simulink model "PowE_lab4_3"  (R2021b)
settings: Solver=VariableStepAuto  StartTime=0.0  StopTime=0.06  RelTol=1e-3
libraries: spsDetailedThyristorLib x2, spsACVoltageSourceLib x1, spsCurrentMeasurementLib x1, spsLinearTransformerLib x1, spsMeanLib x1, spsRMSLib x1, spsSeriesRLCBranchLib x1, spsVoltageMeasurementLib x1, spspowerguiLib x1
settings Model: Creator=shrey  LastModifiedBy=Asus

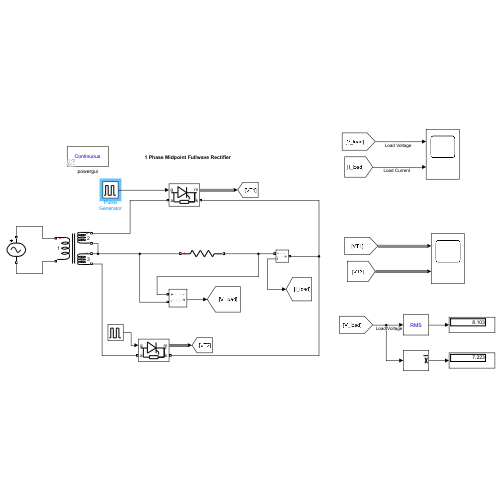
[thumbnail: Simulink's stored preview of the top-level diagram]
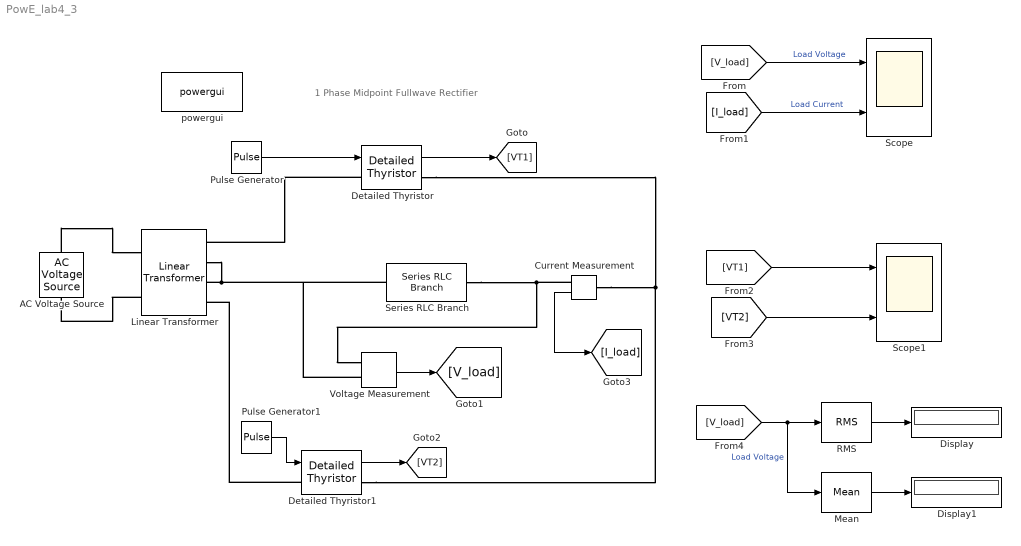
== system PowE_lab4_3 ==
  note: 1 Phase Midpoint Fullwave Rectifier
  AC Voltage Source : spsACVoltageSourceLib/AC Voltage Source  Amplitude=230  Phase=0  Frequency=50  SampleTime=0  Measurements=None  BusType=swing  Pref=10e3  Qref=0  Qmin=-inf  Qmax=+inf
  Current Measurement : spsCurrentMeasurementLib/Current Measurement  PhasorSimulation=off  OutputType=Complex  PSBequivalent=0
  Detailed Thyristor : spsDetailedThyristorLib/Detailed Thyristor  Ron=0.001  Lon=1e-3  Vf=0.8  IL=0.1  Tq=100e-6  IC=0  Rs=500  Cs=250e-9  Measurements=on
      settings: SourceProductBaseCode=PS
  Detailed Thyristor1 : spsDetailedThyristorLib/Detailed Thyristor  Ron=0.001  Lon=1e-3  Vf=0.8  IL=0.1  Tq=100e-6  IC=0  Rs=500  Cs=250e-9  Measurements=on
      settings: SourceProductBaseCode=PS
  Display : Display
  Display1 : Display
  Linear Transformer : spsLinearTransformerLib/Linear Transformer  UNITS=pu  NominalPower=[ 250e6 60 ]  winding1="[ 230  0.002  0.08 ]"  winding2="[ 12  0.002  0.0 ]"  ThreeWindings=on  winding3=[ 12 0.002 0.0 ]  RmLm=[ 500 500 ]  Measurements=None  DataType=off
  Mean : spsMeanLib/Mean  Freq=60  Vinit=0  Ts=0
  Pulse Generator : DiscretePulseGenerator  PulseType=Time based  Period=0.02  PulseWidth=5  PhaseDelay=0.02*(0/360)
  Pulse Generator1 : DiscretePulseGenerator  PulseType=Time based  Period=10  PulseWidth=5  PhaseDelay=0.02*(180)/360
  RMS : spsRMSLib/RMS  TrueRMS=on  Freq=60  RMSInit=120  Ts=0
  Scope : Scope  NumInputPorts=2
  Scope1 : Scope  NumInputPorts=2
  Series RLC Branch : spsSeriesRLCBranchLib/Series RLC Branch  LConnTagsString=__new0  RConnTagsString=__new0  BranchType=R  Resistance=100  Inductance=1e-3  SetiL0=off  InitialCurrent=0  Capacitance=1e-6  Setx0=off  InitialVoltage=0  Measurements=None
  Voltage Measurement : spsVoltageMeasurementLib/Voltage Measurement  PhasorSimulation=off  OutputType=Complex  PSBequivalent=0
  powergui : spspowerguiLib/powergui  Priority=1  SimulationMode=Continuous  SampleTime=50e-6  frequency=60  Iterations=50  frequencyindice=50  Pbase=100e6  ErrMax=1e-4  UnitsV=kV  UnitsW=MW  buscounter=0  FunctionMessages=off  echomessages=off  EnableUseOfTLC=off  CurrentSourceSwitches=off  DisableSnubberDevices=off  DisableRonSwitches=off  DisableVfSwitches=off  DisplayEquations=off  AutomaticDiscreteSolvers=off  SolverType=Tustin/Backward Euler (TBE)  Interpol=off  ExternalGateDelay=off  methode=off  Ts=100  x0status=blocks  SPID=on  SwTol=0  HookPort=off  NonlinearTolerance=1e-4  nMaxIteration=100  ContinueOnMaxIteration=off  RestoreLinks=warning  ResistiveCurrentMeasurement=off  Frange=[0:2:500]  Ylog=off  Xlog=on  ShowGrid=off  save=off  variable=ZData  structure=0  ZoomFFT=off  StartTime=0.0  cycles=1  DisplayStyle=1  fundamental=60  FreqAxis=off  MaxFrequency=1000  frequencyindicesteady=1  RmsSteady=1  display=off
  wires:
  Detailed Thyristor/1 -> [VT1]
  Voltage Measurement/1 -> [V_load]
  Pulse Generator/1 -> Detailed Thyristor/1
  Pulse Generator1/1 -> Detailed Thyristor1/1
  Detailed Thyristor1/1 -> [VT2]
  Current Measurement/1 -> [I_load]
  [V_load] -> Scope/1  "Load Voltage"
  [I_load] -> Scope/2  "Load Current"
  [VT1] -> Scope1/1
  [VT2] -> Scope1/2
  [V_load] -> Mean/1, RMS/1  "Load Voltage"
  RMS/1 -> Display/1
  Mean/1 -> Display1/1
  connections:
  Detailed Thyristor/LConn1 -- Linear Transformer/RConn1
  Linear Transformer/RConn2 -- Voltage Measurement/LConn2 -- Series RLC Branch/LConn1 -- Linear Transformer/RConn3
  Detailed Thyristor1/LConn1 -- Linear Transformer/RConn4
  Series RLC Branch/RConn1 -- Current Measurement/RConn1 -- Voltage Measurement/LConn1
  Current Measurement/LConn1 -- Detailed Thyristor1/RConn1 -- Detailed Thyristor/RConn1
  AC Voltage Source/RConn1 -- Linear Transformer/LConn1
  Linear Transformer/LConn2 -- AC Voltage Source/LConn1
